simulink model "SDME_7"  (R2021b)
settings: Solver=ode1  StartTime=0.0  StopTime=1440  FixedStep=0.1  MaxStep=1e-5  RelTol=1e-3  EnableMultiTasking=on
values from neighbouring files (symbols this model uses):
  Wbatt = 14000*60    (= 840000)    [m_file_SDME_2.m]
settings Model: DisableUpgradeWarningsForVersion=R2015a  Creator=CPES  LastModifiedBy=26295
settings SolverCC: ZeroCrossControl=DisableAll  AlgebraicLoopSolver=TrustRegion  SolverResetMethod=Robust
settings DataIOCC: LimitDataPoints=on  SaveFormat=Array  SignalLoggingSaveFormat=ModelDataLogs  ReturnWorkspaceOutputs=off
settings OptimizationCC: ExpressionDepthLimit=2147483647  LifeSpan=inf
settings DebuggingCC: UnderspecifiedInitializationDetection=Classic  MergeDetectMultiDrivingBlocksExec=none  SolverPrmCheckMsg=warning  FcnCallInpInsideContextMsg=warning  StateNameClashWarn=warning  SFUnexpectedBacktrackingDiag=warning  SFNoUnconditionalDefaultTransitionDiag=warning  SFMachineParentedDataDiag=warning  ArithmeticOperatorsInVariantConditions=warning
settings HardwareCC: ProdBitPerPointer=32  ProdBitPerSizeT=32  ProdBitPerPtrDiffT=32  ProdLargestAtomicFloat=None  ProdIntDivRoundTo=Undefined  ProdEndianess=Unspecified  ProdWordSize=32  ProdHWDeviceType=32-bit Generic
settings ModelReferenceCC: PropagateSignalLabelsOutOfModel=off
settings SFSimCC: SimUseLocalCustomCode=off  CustomCodeUndefinedFunction=UseInterfaceOnly
settings RTWCC: RTWUseLocalCustomCode=off
settings CodeAppCC: StateflowObjectComments=on
settings GRTTargetCC: TargetLangStandard=C89/C90 (ANSI)  CombineOutputUpdateFcns=off  GRTInterface=on
settings ConfigComp: CovMetricSettings=dw  CovSaveCumulativeToWorkspaceVar=on  CovSaveSingleToWorkspaceVar=on  CovExternalEMLEnable=off

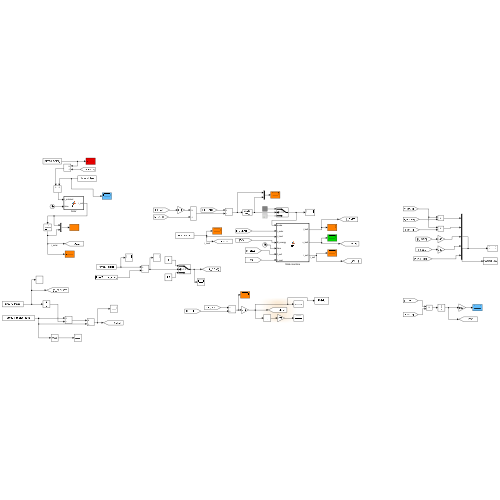
[thumbnail: Simulink's stored preview of the top-level diagram]
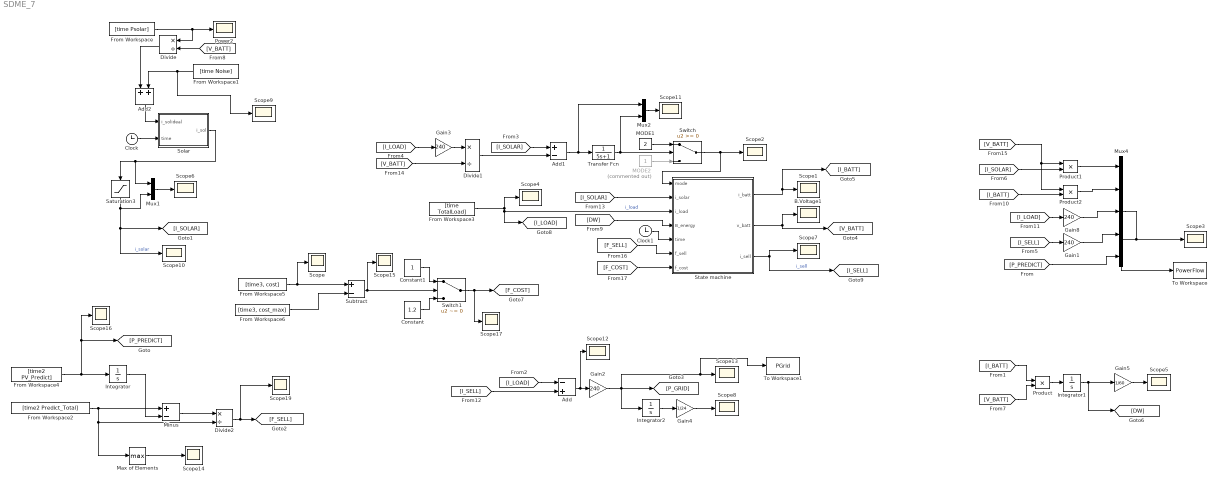
== system SDME_7 ==
  Add : Sum  Inputs=-+
  Add1 : Sum  Inputs=+-
  Add2 : Sum
  B.Voltage1 : Scope
  Clock : Clock
  Clock1 : Clock
  Constant : Constant  Value=1.2
  Constant1 : Constant
  Divide : Product  Inputs=*/
  Divide1 : Product  Inputs=*/
  Divide2 : Product  Inputs=*/
  From Workspace : FromWorkspace  VariableName=[time Psolar]
  From Workspace1 : FromWorkspace  VariableName=[time Noise]
  From Workspace2 : FromWorkspace  VariableName=[time2 Predict_Total]
  From Workspace3 : FromWorkspace  VariableName=[time TotalLoad]
  From Workspace4 : FromWorkspace  VariableName=[time2 PV_Predict]
  From Workspace5 : FromWorkspace  VariableName=[time3, cost]
  From Workspace6 : FromWorkspace  VariableName=[time3, cost_max]
  Gain{1..3,8} (4 alike) : Gain  Gain=240
  Gain4 : Gain  Gain=1/24
  Gain5 : Gain  Gain=1/60
  Integrator : Integrator
  Integrator1 : Integrator  InitialCondition=Wbatt*0+3400*0
  Integrator2 : Integrator
  MODE1 : Constant  Value=2
  MODE2 : Constant  Commented=on
  Max of Elements : MinMax  Function=max
  Minus : Sum  Inputs=+-
  Mux1 : Mux  Inputs=2
  Mux2 : Mux  Inputs=2
  Mux4 : Mux  Inputs=5
  Power2 : Scope
  Product : Product
  Product1 : Product
  Product2 : Product
  Saturation3 : Saturate  UpperLimit=136  LowerLimit=0
  Scope{,1..17,19} (19 alike) : Scope
  Solar : MATLAB Function  TreatAsAtomicUnit=on
  State machine : MATLAB Function  TreatAsAtomicUnit=on
  Subtract : Sum  Inputs=+-
  Switch : Switch
  Switch1 : Switch  Criteria=u2 ~= 0
  To Workspace : ToWorkspace  VariableName=PowerFlow  SaveFormat=Structure With Time  SampleTime=-1
  To Workspace1 : ToWorkspace  VariableName=PGrid  SaveFormat=Structure With Time  SampleTime=-1
  Transfer Fcn : TransferFcn  Denominator=[5 1]
  wires:
  Product/1 -> Integrator1/1
  Mux1/1 -> Scope6/1
  [V_BATT] -> Product/2
  [V_BATT] -> Divide/2
  Integrator1/1 -> [DW], Gain5/1
  From Workspace/1 -> Divide/1, Power2/1
  [I_BATT] -> Product/1
  Saturation3/1 -> Mux1/2, Scope10/1, [I_SOLAR]  "i_solar"
  [I_SOLAR] -> State machine/2(i_solar)
  From Workspace3/1 -> [I_LOAD], State machine/3(i_load), Scope4/1  "i_load"
  [DW] -> State machine/4(B_energy)
  State machine/1(i_batt) -> [I_BATT], Scope1/1
  Add/1 -> Scope12/1, Gain2/1
  State machine/2(v_batt) -> B.Voltage1/1, [V_BATT]
  [I_LOAD] -> Gain8/1
  [I_SELL] -> Gain1/1
  [I_LOAD] -> Add/1
  Gain2/1 -> To Workspace1/1, Scope13/1, Integrator2/1, [P_GRID]
  [I_SELL] -> Add/2
  Divide1/1 -> Add1/2
  [I_LOAD] -> Gain3/1
  Gain3/1 -> Divide1/1
  [V_BATT] -> Divide1/2
  [I_SOLAR] -> Add1/1
  Add1/1 -> Mux2/1, Transfer Fcn/1
  MODE1/1 -> Switch/1
  MODE2/1 -> Switch/3
  Integrator2/1 -> Gain4/1
  Gain4/1 -> Scope8/1
  From Workspace1/1 -> Add2/2, Scope9/1
  Divide/1 -> Add2/1
  Add2/1 -> Solar/1(i_solideal)
  Clock/1 -> Solar/2(time)
  Solar/1(i_sol) -> Mux1/1, Saturation3/1
  Transfer Fcn/1 -> Mux2/2, Switch/2
  Mux2/1 -> Scope11/1
  Gain5/1 -> Scope5/1
  Mux4/1 -> To Workspace/1, Scope3/1
  Product1/1 -> Mux4/1
  Product2/1 -> Mux4/2
  Gain8/1 -> Mux4/3
  Gain1/1 -> Mux4/4
  [I_BATT] -> Product2/2
  [I_SOLAR] -> Product1/2
  [V_BATT] -> Product2/1, Product1/1
  State machine/3(i_sell) -> Scope7/1, [I_SELL]  "i_sell"
  Clock1/1 -> State machine/5(time)
  Switch/1 -> Scope2/1, State machine/1(mode)
  From Workspace4/1 -> Integrator/1, [P_PREDICT], Scope16/1
  [P_PREDICT] -> Mux4/5
  [F_SELL] -> State machine/6(f_sell)
  Integrator/1 -> Minus/2
  From Workspace2/1 -> Max of Elements/1, Divide2/2, Minus/1
  Minus/1 -> Divide2/1
  Divide2/1 -> Scope19/1, [F_SELL]
  Max of Elements/1 -> Scope14/1
  [F_COST] -> State machine/7(f_cost)
  From Workspace5/1 -> Subtract/1, Scope/1
  From Workspace6/1 -> Subtract/2
  Subtract/1 -> Switch1/2, Scope15/1
  Constant/1 -> Switch1/3
  Constant1/1 -> Switch1/1
  Switch1/1 -> [F_COST], Scope17/1

== matlab function SDME_7/State machine ==
  data: mode input; i_solar input; i_batt output; i_load input; B_energy input; v_batt output; i_sell output; time input; f_sell input; f_cost input
function [i_batt, v_batt, i_sell]= fcn(mode, i_solar, i_load, B_energy, time, f_sell, f_cost)
%#codegen

Wbatt=14000*60;
TresholdL = 0;
TresholdH = Wbatt;
I_MAX = 30;

% battery high
Blow=52;
% battery low
Bhigh=57.6;

X=(Bhigh-Blow)/Wbatt;
B_full = 0;
B_empty = 0;

i_sell=0;

v_batt = Blow + X*B_energy;

ratio = v_batt/240;

% Sell Function (from prediction)



% 1: grid zeros
% 2: grid positive
% 3: full power
% 4: night mode

if mode == 1
    i_sell = i_load;
elseif mode == 2
    i_sell = i_solar*ratio*f_sell*f_cost;
%     i_sell = i_solar*ratio*0.2;

elseif mode == 3
    i_sell = I_MAX;
else
    i_sell = 0;
end

% if time > 800  % Only for the last day to finish with fully charged battery
%     i_sell = 0;
% end

i_batt= i_solar - i_sell/ratio;

if (B_energy >= Wbatt) && (i_batt > 0)
    i_batt=0;
    B_full = 1;
else
    B_full = 0;
end

if (B_energy < 0) && (i_batt < 0)
    i_batt=0;
    B_empty = 1;
else
    B_empty = 0;
end

if mode == 3
    if (B_full == 1) || (B_empty == 1)
        i_sell = 0;
    end
end

if B_empty == 1
        i_sell = 0;
end

if B_full == 1
       i_sell = i_solar*ratio;
end

if i_sell > 30
    i_sell = 30;
end



end

== matlab function SDME_7/Solar ==
  data: i_solideal input; time input; i_sol output
function i_sol = fcn(i_solideal,time)
%#codegen

if time < (5*60 + 45) || time > (17*60 +45)
    i_sol = 0;
else
    i_sol = i_solideal;
end
end
